simulink model "ur5bh_Fri"  (R2021b)
settings: Solver=daessc  StartTime=0.0  StopTime=13  FixedStep=1e-4  RelTol=1e-2  AbsTol=1e-2
values from neighbouring files (symbols this model uses):
  Act_Hand = zeros(Phase_Num,1)    [Event2Action.m]
  Act_Lift = zeros(Phase_Num,1)    [Event2Action.m]
  Act_Planner = zeros(Phase_Num,1)    [Event2Action.m]
  Act_Time = zeros(Phase_Num,1)    [Event2Action.m]
  Act_XYZ = zeros(Phase_Num,3)    [Event2Action.m]
  Act_YPR = zeros(Phase_Num,3)    [Event2Action.m]
  maxIter = 200    [Fri_Lancher.m]    (also in ur5bhLancher.m = 50)
undefined symbols (not defined in the file or in its folder): Act_Hand_2, Act_Lift_2, Act_Planner_2, Act_Time_2, Act_XYZ_2, Act_YPR_2, X, Y, Z
libraries: sm_lib x362, nesl_utility x72, robotmaniplib x4, simulink x2
(part 9 of 9)

== system ur5bh_Fri/Dynamic/Subsystem2/wrist_2_joint/wrist_2_link ==
  Inertia : sm_lib/Body Elements/Inertia  InertiaType=Custom  Mass=1.219  MassUnits=kg  CenterOfMass=[0, 0, 0]  CenterOfMassUnits=m  MomentsOfInertia=[0.00255989897604, 0.00255989897604, 0.0021942]  MomentsOfInertiaUnits=kg*m^2  ProductsOfInertia=[0, 0, 0]  ProductsOfInertiaUnits=kg*m^2  GraphicType=None  MarkerShape=Inertia  MarkerSize=20  GraphicVisPropType=SimpleVisualProperties  GraphicDiffuseColor=[0.5 0.5 0.5]  GraphicSpecularColor=[0.5 0.5 0.5 1.0]  GraphicAmbientColor=[0.15 0.15 0.15 1.0]  GraphicEmissiveColor=[0.0 0.0 0.0 1.0]  GraphicShininess=75  GraphicOpacity=1.0
  InertiaOriginTransform : sm_lib/Frames and Transforms/Rigid Transform  TranslationMethod=Cartesian  TranslationStandardOffset=0  TranslationLengthUnit=m  TranslationStandardAxis=+Z  TranslationCartesianOffset=[0, 0, 0.09465]  TranslationROffset=0  TranslationROffsetUnits=m  TranslationZOffset=0  TranslationZOffsetUnits=m  TranslationThetaOffset=0  TranslationThetaOffsetUnits=deg  RotationMethod=RotationSequence  RotationAngleUnits=deg  RotationStandardAxis=+Z  RotationAngle=0.0  RotationArbitraryAxis=[0 0 1]  FollAlignAxisA=+X  BaseAlignAxisA=+Y  FollAlignAxisB=+Y  BaseAlignAxisB=+Z  RotationSequenceAxes=BaseAxes  RotationSequence=XYZ  RotationSequenceAngles=[0, 0, 0]  RotationSequenceAnglesUnits=rad  RotationMatrix=[1 0 0; 0 1 0; 0 0 1]
  ReferenceFrame : sm_lib/Frames and Transforms/Reference Frame
  Visual : sm_lib/Body Elements/File Solid  ExtGeomFileName=ur_description/meshes/ur5/visual/wrist2.stl  UnitType=Custom  ExtGeomFileUnits=m  StepReaderType=HEX  ExportConvexHullGeometry=off  InertiaType=Custom  Mass=0  MassUnits=kg  CenterOfMass=[0, 0, 0]  CenterOfMassUnits=m  MomentsOfInertia=[0, 0, 0]  MomentsOfInertiaUnits=kg*m^2  ProductsOfInertia=[0, 0, 0]  ProductsOfInertiaUnits=kg*m^2  BasedOnType=DensityFromFile  Density=1000  DensityUnits=kg/m^3  DoExposeReferenceFrame=on  SerializedFrames=<Frames/>  GraphicType=FromGeometry  MarkerShape=Sphere  MarkerSize=10  GraphicVisPropType=SimpleVisualProperties  GraphicDiffuseColor=[0.5, 0.5, 0.5]  GraphicSpecularColor=[0.5 0.5 0.5 1.0]  GraphicAmbientColor=[0.15 0.15 0.15 1.0]  GraphicEmissiveColor=[0.0 0.0 0.0 1.0]  GraphicShininess=75  GraphicOpacity=1
  VisualOriginTransform : sm_lib/Frames and Transforms/Rigid Transform  TranslationMethod=Cartesian  TranslationStandardOffset=0  TranslationLengthUnit=m  TranslationStandardAxis=+Z  TranslationCartesianOffset=[0, 0, 0]  TranslationROffset=0  TranslationROffsetUnits=m  TranslationZOffset=0  TranslationZOffsetUnits=m  TranslationThetaOffset=0  TranslationThetaOffsetUnits=deg  RotationMethod=RotationSequence  RotationAngleUnits=deg  RotationStandardAxis=+Z  RotationAngle=0.0  RotationArbitraryAxis=[0 0 1]  FollAlignAxisA=+X  BaseAlignAxisA=+Y  FollAlignAxisB=+Y  BaseAlignAxisB=+Z  RotationSequenceAxes=BaseAxes  RotationSequence=XYZ  RotationSequenceAngles=[0, 0, 0]  RotationSequenceAnglesUnits=rad  RotationMatrix=[1 0 0; 0 1 0; 0 0 1]
  wrist_2_joint_AxisInvTransform : sm_lib/Frames and Transforms/Rigid Transform  TranslationMethod=Cartesian  TranslationStandardOffset=0  TranslationLengthUnit=m  TranslationStandardAxis=+Z  TranslationCartesianOffset=[0, 0, 0]  TranslationROffset=0  TranslationROffsetUnits=m  TranslationZOffset=0  TranslationZOffsetUnits=m  TranslationThetaOffset=0  TranslationThetaOffsetUnits=deg  RotationMethod=ArbitraryAxis  RotationAngleUnits=rad  RotationStandardAxis=+Z  RotationAngle=0  RotationArbitraryAxis=[1, 0, 0]  FollAlignAxisA=+X  BaseAlignAxisA=+Y  FollAlignAxisB=+Y  BaseAlignAxisB=+Z  RotationSequenceAxes=FollowerAxes  RotationSequence=XYX  RotationSequenceAngles=[0 0 0]  RotationSequenceAnglesUnits=deg  RotationMatrix=[1 0 0; 0 1 0; 0 0 1]
  wrist_3_joint_AxisTransform : sm_lib/Frames and Transforms/Rigid Transform  TranslationMethod=Cartesian  TranslationStandardOffset=0  TranslationLengthUnit=m  TranslationStandardAxis=+Z  TranslationCartesianOffset=[0, 0, 0]  TranslationROffset=0  TranslationROffsetUnits=m  TranslationZOffset=0  TranslationZOffsetUnits=m  TranslationThetaOffset=0  TranslationThetaOffsetUnits=deg  RotationMethod=ArbitraryAxis  RotationAngleUnits=rad  RotationStandardAxis=+Z  RotationAngle=1.570796326794897  RotationArbitraryAxis=[-1, 0, 0]  FollAlignAxisA=+X  BaseAlignAxisA=+Y  FollAlignAxisB=+Y  BaseAlignAxisB=+Z  RotationSequenceAxes=FollowerAxes  RotationSequence=XYX  RotationSequenceAngles=[0 0 0]  RotationSequenceAnglesUnits=deg  RotationMatrix=[1 0 0; 0 1 0; 0 0 1]
  wrist_3_joint_OriginTransform : sm_lib/Frames and Transforms/Rigid Transform  TranslationMethod=Cartesian  TranslationStandardOffset=0  TranslationLengthUnit=m  TranslationStandardAxis=+Z  TranslationCartesianOffset=[0, 0, 0.09465]  TranslationROffset=0  TranslationROffsetUnits=m  TranslationZOffset=0  TranslationZOffsetUnits=m  TranslationThetaOffset=0  TranslationThetaOffsetUnits=deg  RotationMethod=RotationSequence  RotationAngleUnits=deg  RotationStandardAxis=+Z  RotationAngle=0.0  RotationArbitraryAxis=[0 0 1]  FollAlignAxisA=+X  BaseAlignAxisA=+Y  FollAlignAxisB=+Y  BaseAlignAxisB=+Z  RotationSequenceAxes=BaseAxes  RotationSequence=XYZ  RotationSequenceAngles=[0, 0, 0]  RotationSequenceAnglesUnits=rad  RotationMatrix=[1 0 0; 0 1 0; 0 0 1]
  F : PMIOPort  Side=Left
  F1 : PMIOPort  Port=2  Side=Right
  connections:
  Inertia/RConn1 -- InertiaOriginTransform/RConn1
  ReferenceFrame/RConn1 -- InertiaOriginTransform/LConn1 -- VisualOriginTransform/LConn1 -- wrist_2_joint_AxisInvTransform/LConn1 -- wrist_3_joint_OriginTransform/LConn1
  Visual/RConn1 -- VisualOriginTransform/RConn1
  wrist_2_joint_AxisInvTransform/RConn1 -- F/RConn1
  wrist_3_joint_AxisTransform/RConn1 -- F1/RConn1
  wrist_3_joint_AxisTransform/LConn1 -- wrist_3_joint_OriginTransform/RConn1

== system ur5bh_Fri/Dynamic/Subsystem2/wrist_3_joint/wrist_3_link ==
  Inertia : sm_lib/Body Elements/Inertia  InertiaType=Custom  Mass=0.1879  MassUnits=kg  CenterOfMass=[0, 0, 0]  CenterOfMassUnits=m  MomentsOfInertia=[8.469589112163001e-05, 8.469589112163001e-05, 0.0001321171875]  MomentsOfInertiaUnits=kg*m^2  ProductsOfInertia=[0, 0, 0]  ProductsOfInertiaUnits=kg*m^2  GraphicType=None  MarkerShape=Inertia  MarkerSize=20  GraphicVisPropType=SimpleVisualProperties  GraphicDiffuseColor=[0.5 0.5 0.5]  GraphicSpecularColor=[0.5 0.5 0.5 1.0]  GraphicAmbientColor=[0.15 0.15 0.15 1.0]  GraphicEmissiveColor=[0.0 0.0 0.0 1.0]  GraphicShininess=75  GraphicOpacity=1.0
  InertiaOriginTransform : sm_lib/Frames and Transforms/Rigid Transform  TranslationMethod=Cartesian  TranslationStandardOffset=0  TranslationLengthUnit=m  TranslationStandardAxis=+Z  TranslationCartesianOffset=[0, 0.06505, 0]  TranslationROffset=0  TranslationROffsetUnits=m  TranslationZOffset=0  TranslationZOffsetUnits=m  TranslationThetaOffset=0  TranslationThetaOffsetUnits=deg  RotationMethod=RotationSequence  RotationAngleUnits=deg  RotationStandardAxis=+Z  RotationAngle=0.0  RotationArbitraryAxis=[0 0 1]  FollAlignAxisA=+X  BaseAlignAxisA=+Y  FollAlignAxisB=+Y  BaseAlignAxisB=+Z  RotationSequenceAxes=BaseAxes  RotationSequence=XYZ  RotationSequenceAngles=[1.570796326794897, 0, 0]  RotationSequenceAnglesUnits=rad  RotationMatrix=[1 0 0; 0 1 0; 0 0 1]
  ReferenceFrame : sm_lib/Frames and Transforms/Reference Frame
  Visual : sm_lib/Body Elements/File Solid  ExtGeomFileName=ur_description/meshes/ur5/visual/wrist3.stl  UnitType=Custom  ExtGeomFileUnits=m  StepReaderType=HEX  ExportConvexHullGeometry=off  InertiaType=Custom  Mass=0  MassUnits=kg  CenterOfMass=[0, 0, 0]  CenterOfMassUnits=m  MomentsOfInertia=[0, 0, 0]  MomentsOfInertiaUnits=kg*m^2  ProductsOfInertia=[0, 0, 0]  ProductsOfInertiaUnits=kg*m^2  BasedOnType=DensityFromFile  Density=1000  DensityUnits=kg/m^3  DoExposeReferenceFrame=on  SerializedFrames=<Frames/>  GraphicType=FromGeometry  MarkerShape=Sphere  MarkerSize=10  GraphicVisPropType=SimpleVisualProperties  GraphicDiffuseColor=[0.5, 0.5, 0.5]  GraphicSpecularColor=[0.5 0.5 0.5 1.0]  GraphicAmbientColor=[0.15 0.15 0.15 1.0]  GraphicEmissiveColor=[0.0 0.0 0.0 1.0]  GraphicShininess=75  GraphicOpacity=1
  VisualOriginTransform : sm_lib/Frames and Transforms/Rigid Transform  TranslationMethod=Cartesian  TranslationStandardOffset=0  TranslationLengthUnit=m  TranslationStandardAxis=+Z  TranslationCartesianOffset=[0, 0, 0]  TranslationROffset=0  TranslationROffsetUnits=m  TranslationZOffset=0  TranslationZOffsetUnits=m  TranslationThetaOffset=0  TranslationThetaOffsetUnits=deg  RotationMethod=RotationSequence  RotationAngleUnits=deg  RotationStandardAxis=+Z  RotationAngle=0.0  RotationArbitraryAxis=[0 0 1]  FollAlignAxisA=+X  BaseAlignAxisA=+Y  FollAlignAxisB=+Y  BaseAlignAxisB=+Z  RotationSequenceAxes=BaseAxes  RotationSequence=XYZ  RotationSequenceAngles=[0, 0, 0]  RotationSequenceAnglesUnits=rad  RotationMatrix=[1 0 0; 0 1 0; 0 0 1]
  ee_fixed_joint_OriginTransform : sm_lib/Frames and Transforms/Rigid Transform  TranslationMethod=Cartesian  TranslationStandardOffset=0  TranslationLengthUnit=m  TranslationStandardAxis=+Z  TranslationCartesianOffset=[0, 0.0823, 0]  TranslationROffset=0  TranslationROffsetUnits=m  TranslationZOffset=0  TranslationZOffsetUnits=m  TranslationThetaOffset=0  TranslationThetaOffsetUnits=deg  RotationMethod=RotationSequence  RotationAngleUnits=deg  RotationStandardAxis=+Z  RotationAngle=0.0  RotationArbitraryAxis=[0 0 1]  FollAlignAxisA=+X  BaseAlignAxisA=+Y  FollAlignAxisB=+Y  BaseAlignAxisB=+Z  RotationSequenceAxes=BaseAxes  RotationSequence=XYZ  RotationSequenceAngles=[0, 0, 1.570796326794897]  RotationSequenceAnglesUnits=rad  RotationMatrix=[1 0 0; 0 1 0; 0 0 1]
  wrist_3_joint_AxisInvTransform : sm_lib/Frames and Transforms/Rigid Transform  TranslationMethod=Cartesian  TranslationStandardOffset=0  TranslationLengthUnit=m  TranslationStandardAxis=+Z  TranslationCartesianOffset=[0, 0, 0]  TranslationROffset=0  TranslationROffsetUnits=m  TranslationZOffset=0  TranslationZOffsetUnits=m  TranslationThetaOffset=0  TranslationThetaOffsetUnits=deg  RotationMethod=ArbitraryAxis  RotationAngleUnits=rad  RotationStandardAxis=+Z  RotationAngle=1.570796326794897  RotationArbitraryAxis=[-1, 0, 0]  FollAlignAxisA=+X  BaseAlignAxisA=+Y  FollAlignAxisB=+Y  BaseAlignAxisB=+Z  RotationSequenceAxes=FollowerAxes  RotationSequence=XYX  RotationSequenceAngles=[0 0 0]  RotationSequenceAnglesUnits=deg  RotationMatrix=[1 0 0; 0 1 0; 0 0 1]
  F : PMIOPort  Side=Left
  F1 : PMIOPort  Port=2  Side=Right
  connections:
  Inertia/RConn1 -- InertiaOriginTransform/RConn1
  ReferenceFrame/RConn1 -- InertiaOriginTransform/LConn1 -- wrist_3_joint_AxisInvTransform/LConn1 -- ee_fixed_joint_OriginTransform/LConn1 -- VisualOriginTransform/LConn1
  Visual/RConn1 -- VisualOriginTransform/RConn1
  ee_fixed_joint_OriginTransform/RConn1 -- F1/RConn1
  wrist_3_joint_AxisInvTransform/RConn1 -- F/RConn1

== matlab function ur5bh_Fri/Planner/Trajectory Planner/IK_Linear/MATLAB Function ==
  data: xyz input; Pose output; ypr input
function Pose=GetPose(xyz,ypr)
R=eul2rotm(ypr)*eul2rotm([-pi/2 -pi/2 0]);
Pose=[R xyz;[0 0 0 1]];
end

== matlab function ur5bh_Fri/Planner/Trajectory Planner/IK_Linear/MATLAB Function1 ==
  data: StartConfig input; Path output; FinalConfig input; maxIter input
function Path = fcn(StartConfig,FinalConfig,maxIter)

Path=zeros(1206,1)*0.0;
Path(1,1)=maxIter;
for i=1:maxIter
    for j=1:6
    Path(i*6+j,1)=StartConfig(j)+(1-exp(-(i-1)/(maxIter-1)))*(FinalConfig(j)-StartConfig(j));
    end
end

== matlab function ur5bh_Fri/Planner/Trajectory Planner/Singal Select ==
  data: Act_Planner input; y output; RRT input size=maxIter*6+6; IK_Linear input size=maxIter*6+6; Linear input; None input size=maxIter*6+6
function y = fcn(Act_Planner,RRT,IK_Linear,Linear,None)

switch Act_Planner
    case 0
        y=None;
    case 1
        y=RRT;
    case 2
        y=IK_Linear;
    case 3
        y=Linear;
    otherwise
        y=None;
end

== matlab function ur5bh_Fri/Planner/Trajectory Planner/None/MATLAB Function1 ==
  data: StartConfig input; Path output; maxIter input
function Path = fcn(StartConfig,maxIter)

Path=zeros(1206,1)*0.0;
Path(1)=maxIter;
for i=1:maxIter
    for j=1:6
    Path(i*6+j)=StartConfig(j);
    end
end

== matlab function ur5bh_Fri/Dynamic/Subsystem/MATLAB Function ==
  data: LiftCom input; r output
function r = fcn(LiftCom)
if LiftCom==0
    r=0.045;
else
    r=0.00001;
end

== matlab function ur5bh_Fri/Dynamic/hand/Subsystem/MATLAB Function ==
  data: LiftCom input; r output
function r = fcn(LiftCom)
if LiftCom==1
    r=0.045;
else
    r=0.00001;
end

== matlab function ur5bh_Fri/Dynamic/Subsystem/MATLAB Function1 ==
  data: LiftCom input; r output
function r = fcn(LiftCom)
if LiftCom==2
    r=0.045;
else
    r=0.00001;
end

== matlab function ur5bh_Fri/Planner1/Trajectory Planner/IK_Linear1/MATLAB Function1 ==
  data: StartConfig input; ypr input; xyz input; Path output; maxIter input
function Path = fcn(StartConfig,ypr,xyz,maxIter)
FinalConfig=[xyz(1) xyz(2) xyz(3) ypr(1) ypr(2) ypr(3)];
Path=zeros(1206,1)*0.0;
Path(1,1)=maxIter;
for i=1:maxIter
    for j=1:6
    Path(i*6+j,1)=StartConfig(j)+(1-exp(-(i-1)/(maxIter-1)))*(FinalConfig(j)-StartConfig(j));
    end
end

== matlab function ur5bh_Fri/Joint Controller2/MATLAB Function1 ==
  data: LiftCom input; FExt output
function FExt= fcn(LiftCom)

FExt=zeros(6,20);
if LiftCom==1
    FExt(6,10)=1;
end

== matlab function ur5bh_Fri/MATLAB Function ==
  data: FingerTau1 output; HandCom1 input; FingerTau2 output; HandCom2 input
function [FingerTau1,FingerTau2] = fcn(HandCom1,HandCom2)
if HandCom1==1
    FingerTau1=300*[1 1 1];
else
    FingerTau1=-300*[1 1 1];
end
if HandCom2==1
    FingerTau2=300*[1 1 1];
else
    FingerTau2=-300*[1 1 1];
end
end

== matlab function ur5bh_Fri/Joint Controller2/PD ==
  data: qd input size=6; wd input; w input; q input size=6; JointAcc output size=6
function JointAcc = PDControl(qd,wd,w,q)
kq=10;
kw=8;
JointAcc=zeros(6,1);
for i=1:6
    JointAcc(i)=kq*(qd(i)-q(i))+kw*(wd(i)-w(i));
end
end

== matlab function ur5bh_Fri/Planner1/Action Commander ==
  settings: updateMethod=DISCRETE
  data: t input; ArmBase input; Planner_Pulse output; Com_Planner output; Com_XYZ output; Com_YPR output; Com_Hand output; Com_Time output; EventCycle data_store_memory; TimeStamp data_store_memory; Act_Hand input; Act_Planner input; Act_XYZ input; Act_YPR input; Act_Time input; Act_Lift input; Com_Lift output
function [Planner_Pulse,Com_Planner,Com_XYZ,Com_YPR,Com_Hand,Com_Time,Com_Lift] = PlannerTrigger(t,ArmBase,Act_Hand,Act_Planner,Act_XYZ,Act_YPR,Act_Time,Act_Lift)

global TimeStamp;
global EventCycle;

PhaseCount=size(Act_Time,1);
if (t>Act_Time(EventCycle))&&((EventCycle+1)<=PhaseCount)
    EventCycle=EventCycle+1;
    Planner_Pulse=1;
else
    Planner_Pulse=-1;
end

if t<Act_Time(PhaseCount)&&t>Act_Time(1)
    Com_Time=Act_Time(EventCycle)-Act_Time(EventCycle-1);
    Shift_t=t-Act_Time(EventCycle-1);
elseif t<Act_Time(1)
    Com_Time=Act_Time(1);
    Shift_t=t;
else
    Com_Time=10000;
    Shift_t=t;
end

if EventCycle==0
    Com_Hand=0;
    Com_XYZ=[0; 0; 0];
    Com_Planner=0;
    Com_YPR=[0 0 0];
    Com_Lift=0;
else
    Com_Hand=Act_Hand(EventCycle);
    Com_XYZ=Act_XYZ(EventCycle,:).'-ArmBase;
    Com_Planner=Act_Planner(EventCycle);
    Com_YPR=Act_YPR(EventCycle,:);
    Com_Lift=Act_Lift(EventCycle);
end


TimeStamp=floor(Shift_t*1000);

== matlab function ur5bh_Fri/Planner1/Trajectory Planner/IK_Linear/MATLAB Function ==
  data: xyz input; Pose output; ypr input
function Pose=GetPose(xyz,ypr)
R=eul2rotm(ypr)*eul2rotm([-pi/2 -pi/2 0]);
Pose=[R xyz;[0 0 0 1]];
end

== matlab function ur5bh_Fri/Planner1/Trajectory Planner/IK_Linear/MATLAB Function1 ==
  data: StartConfig input; Path output; FinalConfig input; maxIter input
function Path = fcn(StartConfig,FinalConfig,maxIter)

Path=zeros(1206,1)*0.0;
Path(1,1)=maxIter;
for i=1:maxIter
    for j=1:6
    Path(i*6+j,1)=StartConfig(j)+(1-exp(-(i-1)/(maxIter-1)))*(FinalConfig(j)-StartConfig(j));
    end
end

== matlab function ur5bh_Fri/Planner1/Trajectory Planner/None/MATLAB Function1 ==
  data: StartConfig input; Path output; maxIter input
function Path = fcn(StartConfig,maxIter)

Path=zeros(1206,1)*0.0;
Path(1)=maxIter;
for i=1:maxIter
    for j=1:6
    Path(i*6+j)=StartConfig(j);
    end
end

== matlab function ur5bh_Fri/Planner1/Trajectory Planner/RRT Planner/MATLAB Function ==
  data: Q input; xyz input; RRTInput output; ypr input; maxIter input
function RRTInput=Encoder(Q,xyz,ypr,maxIter)
    RRTInput=[Q(1) Q(2) Q(3) Q(4) Q(5) Q(6) ypr(1) ypr(2) ypr(3) xyz(1) xyz(2) xyz(3) maxIter];
end

== matlab function ur5bh_Fri/Planner1/Trajectory Planner/Singal Select ==
  data: Act_Planner input; y output; RRT input size=maxIter*6+6; IK_Linear input size=maxIter*6+6; Linear input; None input size=maxIter*6+6
function y = fcn(Act_Planner,RRT,IK_Linear,Linear,None)

switch Act_Planner
    case 0
        y=None;
    case 1
        y=RRT;
    case 2
        y=IK_Linear;
    case 3
        y=Linear;
    otherwise
        y=None;
end

== matlab function ur5bh_Fri/Planner1/Trajectroies to desire q ==
  data: timeStamp input; T input; desireQ output size=6; Tras input double size=maxIter*6+6
function desireQ = FollowTra(timeStamp,T,Tras)
% col=Trajectories(2);
% Frequency=100; %100HZ
Frequency=floor((Tras(1,1)+1)/T);
step=min(ceil(timeStamp/1000*Frequency),Tras(1,1));
step=max(step,1);
desireQ=zeros(6,1);
for i=1:6
    desireQ(i)=Tras(step*6+i,1);
end
end

== matlab function ur5bh_Fri/Planner/Trajectory Planner/Linear/MATLAB Function1 ==
  data: StartConfig input; ypr input; xyz input; Path output; maxIter input
function Path = fcn(StartConfig,ypr,xyz,maxIter)
FinalConfig=[xyz(1) xyz(2) xyz(3) ypr(1) ypr(2) ypr(3)];
Path=zeros(1206,1)*0.0;
Path(1,1)=maxIter;
for i=1:maxIter
    for j=1:6
    Path(i*6+j,1)=StartConfig(j)+(1-exp(-(i-1)/(maxIter-1)))*(FinalConfig(j)-StartConfig(j));
    end
end

== matlab function ur5bh_Fri/Planner/Trajectroies to desire q ==
  data: timeStamp input; T input; desireQ output size=6; Tras input double size=maxIter*6+6
function desireQ = FollowTra(timeStamp,T,Tras)
% col=Trajectories(2);
% Frequency=100; %100HZ
Frequency=floor((Tras(1,1)+1)/T);
step=min(ceil(timeStamp/1000*Frequency),Tras(1,1));
step=max(step,1);
desireQ=zeros(6,1);
for i=1:6
    desireQ(i)=Tras(step*6+i,1);
end
end

== matlab function ur5bh_Fri/Joint Controller/PD ==
  data: qd input size=6; wd input; w input; q input size=6; JointAcc output size=6
function JointAcc = PDControl(qd,wd,w,q)
kq=10;
kw=8;
JointAcc=zeros(6,1);
for i=1:6
    JointAcc(i)=kq*(qd(i)-q(i))+kw*(wd(i)-w(i));
end
end

== matlab function ur5bh_Fri/Joint Controller/MATLAB Function ==
  data: q input; desireQ input; desireQ2 output
function desireQ2 = SaturateQ(q,desireQ)
desireQ2=desireQ;
for i=1:6
    if abs(desireQ(i)-q(i))>pi
        desireQ2(i)=desireQ(i)-2*pi;
    end
end

== matlab function ur5bh_Fri/Planner/Action Commander ==
  settings: updateMethod=DISCRETE
  data: t input; ArmBase input; Planner_Pulse output; Com_Planner output; Com_XYZ output; Com_YPR output; Com_Hand output; Com_Time output; EventCycle data_store_memory; TimeStamp data_store_memory; Act_Hand input; Act_Planner input; Act_XYZ input; Act_YPR input; Act_Time input; Act_Lift input; Com_Lift output
function [Planner_Pulse,Com_Planner,Com_XYZ,Com_YPR,Com_Hand,Com_Time,Com_Lift] = PlannerTrigger(t,ArmBase,Act_Hand,Act_Planner,Act_XYZ,Act_YPR,Act_Time,Act_Lift)

global TimeStamp;
global EventCycle;

PhaseCount=size(Act_Time,1);
if (t>Act_Time(EventCycle))&&((EventCycle+1)<=PhaseCount)
    EventCycle=EventCycle+1;
    Planner_Pulse=1;
else
    Planner_Pulse=-1;
end

if t<Act_Time(PhaseCount)&&t>Act_Time(1)
    Com_Time=Act_Time(EventCycle)-Act_Time(EventCycle-1);
    Shift_t=t-Act_Time(EventCycle-1);
elseif t<Act_Time(1)
    Com_Time=Act_Time(1);
    Shift_t=t;
else
    Com_Time=10000;
    Shift_t=t;
end

if EventCycle==0
    Com_Hand=0;
    Com_XYZ=[0; 0; 0];
    Com_Planner=0;
    Com_YPR=[0 0 0];
    Com_Lift=0;
else
    Com_Hand=Act_Hand(EventCycle);
    Com_XYZ=Act_XYZ(EventCycle,:).'-ArmBase;
    Com_Planner=Act_Planner(EventCycle);
    Com_YPR=Act_YPR(EventCycle,:);
    Com_Lift=Act_Lift(EventCycle);
end


TimeStamp=floor(Shift_t*1000);

== matlab function ur5bh_Fri/Joint Controller2/MATLAB Function ==
  data: q input; desireQ input; desireQ2 output
function desireQ2 = SaturateQ(q,desireQ)
desireQ2=desireQ;
for i=1:6
    if abs(desireQ(i)-q(i))>pi
        desireQ2(i)=desireQ(i)-2*pi;
    end
end

== matlab function ur5bh_Fri/Joint Controller/MATLAB Function1 ==
  data: LiftCom input; FExt output
function FExt= fcn(LiftCom)

FExt=zeros(6,20);
if LiftCom==1
    FExt(6,10)=1;
end

== matlab function ur5bh_Fri/Planner/Trajectory Planner/RRT Planner/MATLAB Function ==
  data: Q input; xyz input; RRTInput output; ypr input; maxIter input
function RRTInput=Encoder(Q,xyz,ypr,maxIter)
    RRTInput=[Q(1) Q(2) Q(3) Q(4) Q(5) Q(6) ypr(1) ypr(2) ypr(3) xyz(1) xyz(2) xyz(3) maxIter];
end
